simulink model "part4"  (R2014a)
settings: Solver=ode45  StartTime=0.0  StopTime=10.0  RelTol=1e-3
settings Model: Creator=SuperUser  LastModifiedBy=SuperUser

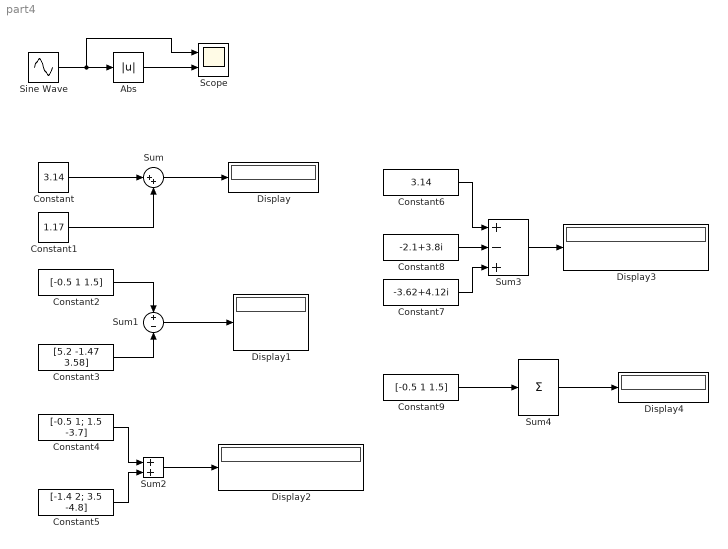
== system part4 ==
  Abs : Abs
  Constant : Constant  Value=3.14
  Constant1 : Constant  Value=1.17
  Constant2 : Constant  Value=[-0.5 1 1.5]
  Constant3 : Constant  Value=[5.2 -1.47 3.58]
  Constant4 : Constant  Value=[-0.5 1; 1.5 -3.7]
  Constant5 : Constant  Value=[-1.4 2; 3.5 -4.8]
  Constant6 : Constant  Value=3.14
  Constant7 : Constant  Value=-3.62+4.12i
  Constant8 : Constant  Value=-2.1+3.8i
  Constant9 : Constant  Value=[-0.5 1 1.5]
  Display{,1..4} (5 alike) : Display
  Scope : Scope  NumInputPorts=2
      settings: YMin=-5~-5  YMax=5~5
  Sine Wave : Sin  SampleTime=0
  Sum : Sum  Inputs=|++
  Sum1 : Sum  Inputs=+-
  Sum2 : Sum
  Sum3 : Sum  Inputs=+-+
  Sum4 : Sum  Inputs=1
  wires:
  Sine Wave/1 -> Scope/1, Abs/1
  Abs/1 -> Scope/2
  Constant/1 -> Sum/1
  Constant1/1 -> Sum/2
  Sum/1 -> Display/1
  Constant2/1 -> Sum1/1
  Constant3/1 -> Sum1/2
  Sum1/1 -> Display1/1
  Constant4/1 -> Sum2/1
  Constant5/1 -> Sum2/2
  Sum2/1 -> Display2/1
  Constant6/1 -> Sum3/1
  Sum3/1 -> Display3/1
  Constant7/1 -> Sum3/3
  Constant8/1 -> Sum3/2
  Constant9/1 -> Sum4/1
  Sum4/1 -> Display4/1
